simulink model "LQR_Active_suspension"  (R2024b)
settings: Solver=VariableStepAuto  StartTime=0.0  StopTime=10.0  RelTol=1e-3
values from neighbouring files (symbols this model uses):
  A = [ 0 1 0 -1 ... (first row only)    [param.m]
  a = 0.4    [param.m]
  B = [0  0 ... (first row only)    [param.m]
  C = [ 1 0 0 0 ... (first row only)    [param.m]
  D = [0 0 ... (first row only)    [param.m]
  F = 3    [param.m]
  K = lqr( A, B(:,2), Q, R )    [param.m]
libraries: eeGeneralControl x1
settings Model: Creator=rob  LastModifiedBy=rob

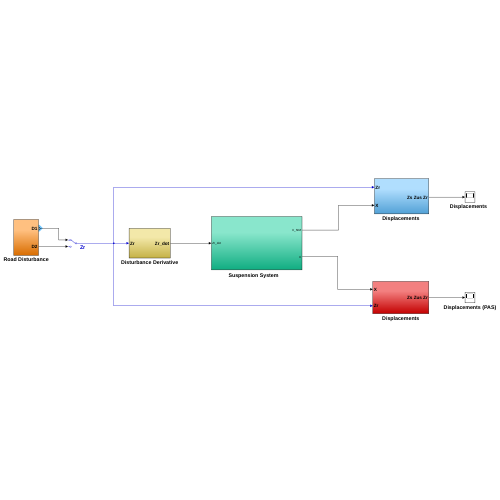
[thumbnail: Simulink's stored preview of the top-level diagram]
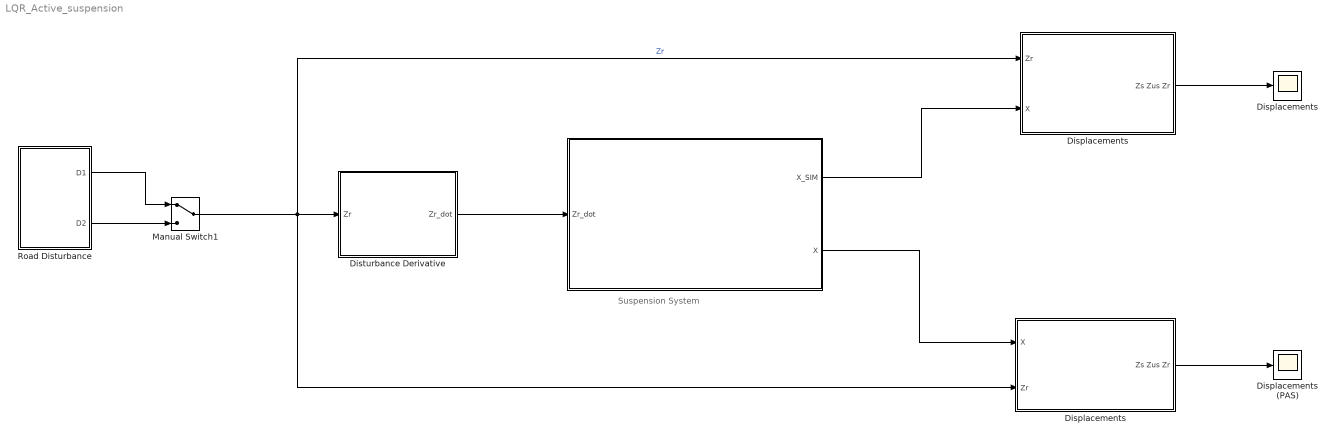
== system LQR_Active_suspension ==
  note: Suspension System
  " " : Subsystem
  Displacements : Subsystem
  "Displacements " : Subsystem
  "Displacements  " : Scope
  Displacements (PAS) : Scope
  Disturbance Derivative : Subsystem
  Manual Switch1 : ManualSwitch
  Road Disturbance : Subsystem
  wires:
  "Displacements "/1(Zs Zus Zr) -> "Displacements  "/1
  Road Disturbance/2(D2) -> Manual Switch1/2
  Road Disturbance/1(D1) -> Manual Switch1/1
  Manual Switch1/1 -> Disturbance Derivative/1(Zr), Displacements/2(Zr), "Displacements "/1(Zr)  "Zr"
  Displacements/1(Zs Zus Zr) -> Displacements (PAS)/1
  " "/2(X) -> Displacements/1(X)
  " "/1(X_SIM) -> "Displacements "/2(X)
  Disturbance Derivative/1(Zr_dot) -> " "/1(Zr_dot)

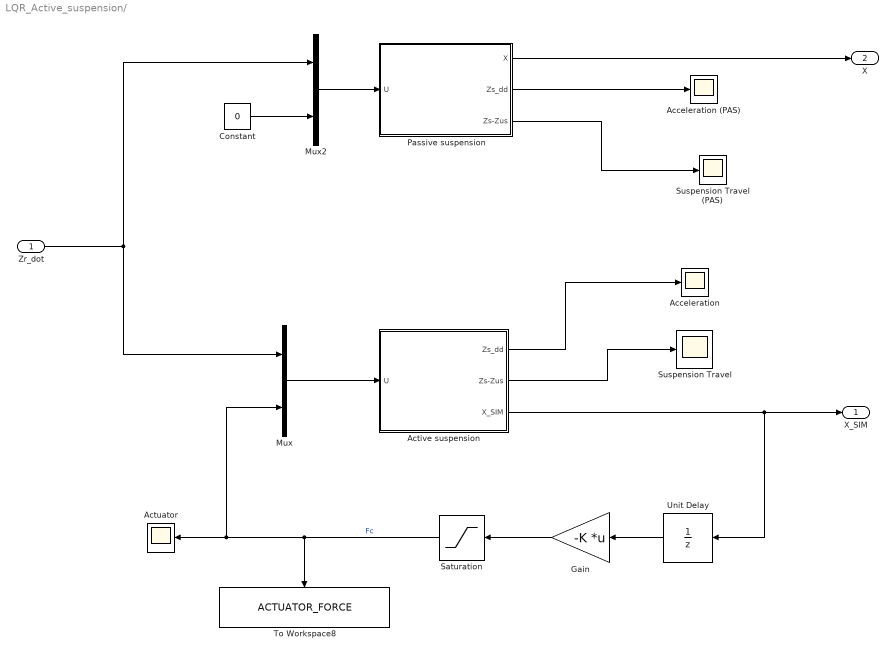
== system LQR_Active_suspension/  ==
  Zr_dot : Inport
  Acceleration : Scope
  Acceleration (PAS) : Scope
  Active suspension : Subsystem
  Actuator : Scope
  Constant : Constant  Value=0
  "Gain " : Gain  Gain=-K  Multiplication=Matrix(K*u)
  Mux : Mux  Inputs=2
  Mux2 : Mux  Inputs=2
  Passive suspension : Subsystem
  Saturation : Saturate  UpperLimit=45000  LowerLimit=-45000
  Suspension Travel : Scope
  Suspension Travel (PAS) : Scope
  To Workspace8 : ToWorkspace  VariableName=ACTUATOR_FORCE  SaveFormat=Timeseries  SampleTime=-1
  Unit Delay : UnitDelay  SampleTime=-1  HasFrameUpgradeWarning=on
  X_SIM : Outport
  X : Outport  Port=2
  wires:
  Active suspension/1(Zs_dd) -> Acceleration/1
  Mux/1 -> Active suspension/1(U)
  Zr_dot/1 -> Mux/1, Mux2/1
  Unit Delay/1 -> "Gain "/1
  Constant/1 -> Mux2/2
  Saturation/1 -> Mux/2, Actuator/1, To Workspace8/1  "Fc"
  "Gain "/1 -> Saturation/1
  Active suspension/3(X_SIM) -> X_SIM/1, Unit Delay/1
  Mux2/1 -> Passive suspension/1(U)
  Passive suspension/2(Zs_dd) -> Acceleration (PAS)/1
  Active suspension/2(Zs-Zus) -> Suspension Travel/1
  Passive suspension/3(Zs-Zus) -> Suspension Travel (PAS)/1
  Passive suspension/1(X) -> X/1

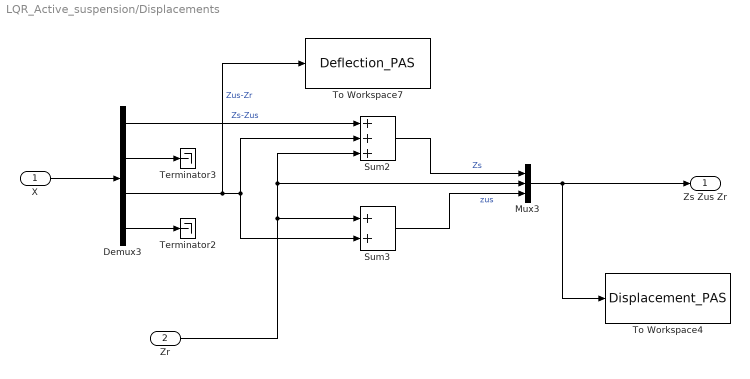
== system LQR_Active_suspension/Displacements ==
  X : Inport
  Zr : Inport  Port=2
  Demux3 : Demux
  Mux3 : Mux  Inputs=3
  Sum2 : Sum  Inputs=+++
  Sum3 : Sum
  Terminator2 : Terminator
  Terminator3 : Terminator
  To Workspace4 : ToWorkspace  VariableName=Displacement_PAS  SaveFormat=Timeseries  SampleTime=-1
  To Workspace7 : ToWorkspace  VariableName=Deflection_PAS  SaveFormat=Timeseries  SampleTime=-1
  Zs Zus Zr : Outport
  wires:
  Demux3/2 -> Terminator3/1
  Demux3/4 -> Terminator2/1
  Demux3/1 -> Sum2/1  "Zs-Zus"
  Demux3/3 -> To Workspace7/1, Sum3/2, Sum2/2  "Zus-Zr"
  Sum2/1 -> Mux3/1  "Zs"
  Sum3/1 -> Mux3/3  "zus"
  Mux3/1 -> Zs Zus Zr/1, To Workspace4/1
  Zr/1 -> Sum3/1, Mux3/2, Sum2/3
  X/1 -> Demux3/1

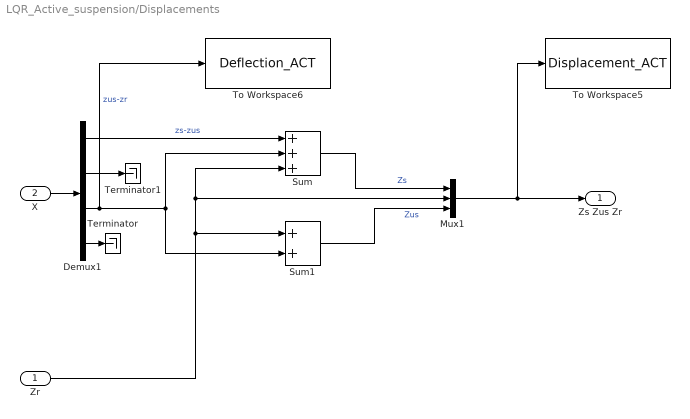
== system LQR_Active_suspension/Displacements  ==
  Zr : Inport
  X : Inport  Port=2
  Demux1 : Demux
  Mux1 : Mux  Inputs=3
  Sum : Sum  Inputs=+++
  Sum1 : Sum
  Terminator : Terminator
  Terminator1 : Terminator
  To Workspace5 : ToWorkspace  VariableName=Displacement_ACT  SaveFormat=Timeseries  SampleTime=-1
  To Workspace6 : ToWorkspace  VariableName=Deflection_ACT  SaveFormat=Timeseries  SampleTime=-1
  Zs Zus Zr : Outport
  wires:
  X/1 -> Demux1/1
  Demux1/2 -> Terminator1/1
  Demux1/4 -> Terminator/1
  Demux1/1 -> Sum/1  "zs-zus"
  Demux1/3 -> To Workspace6/1, Sum1/2, Sum/2  "zus-zr"
  Sum/1 -> Mux1/1  "Zs"
  Sum1/1 -> Mux1/3  "Zus"
  Mux1/1 -> Zs Zus Zr/1, To Workspace5/1
  Zr/1 -> Sum1/1, Mux1/2, Sum/3

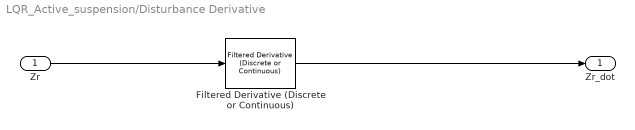
== system LQR_Active_suspension/Disturbance Derivative ==
  Zr : Inport
  Filtered Derivative (Discrete or Continuous) : eeGeneralControl/Filtered Derivative (Discrete or Continuous)  K=1  T=0.015  B=inf  A=-inf  minRatio=10  init_option=Inherited from block input  x0=0  Ts=-1
      settings: LibrarySourceBlock=|
      | ee_sl_lib/General Control/Filtered Derivative
      | (Discrete or Continuous)
  Zr_dot : Outport
  wires:
  Zr/1 -> Filtered Derivative (Discrete or Continuous)/1
  Filtered Derivative (Discrete or Continuous)/1 -> Zr_dot/1

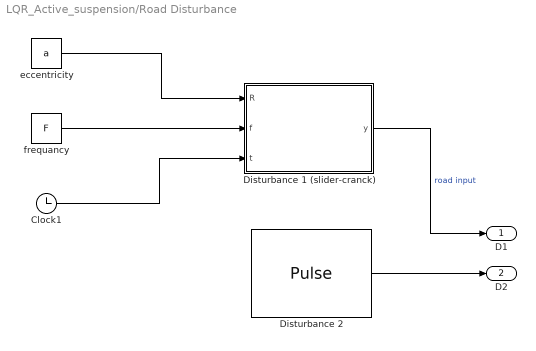
== system LQR_Active_suspension/Road Disturbance ==
  Clock1 : Clock
      settings: Decimation=Sim_Time
  Disturbance 1 (slider-cranck) : MATLAB Function  TreatAsAtomicUnit=on
  Disturbance 2 : DiscretePulseGenerator  PulseType=Time based  Amplitude=0.1  Period=6  PulseWidth=50  PhaseDelay=.1
  eccentricity : Constant  Value=a
  frequancy : Constant  Value=F
  D1 : Outport
  D2 : Outport  Port=2
  wires:
  Disturbance 2/1 -> D2/1
  eccentricity/1 -> Disturbance 1 (slider-cranck)/1(R)
  frequancy/1 -> Disturbance 1 (slider-cranck)/2(f)
  Clock1/1 -> Disturbance 1 (slider-cranck)/3(t)
  Disturbance 1 (slider-cranck)/1(y) -> D1/1  "road input"

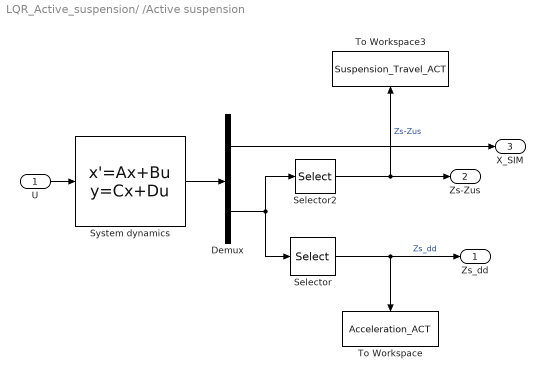
== system LQR_Active_suspension/ /Active suspension ==
  U : Inport
  Demux : Demux  Outputs=[4 2]
  Selector : Selector  InputPortWidth=2  IndexOptions=Index vector (dialog)  Indices=[2]  OutputSizes=1
  Selector2 : Selector  InputPortWidth=2  IndexOptions=Index vector (dialog)  Indices=[1]  OutputSizes=1
  System dynamics : StateSpace  A=A  B=B  C=cat(1,eye(4), C)  D=D  InitialCondition=0
  To Workspace : ToWorkspace  VariableName=Acceleration_ACT  SaveFormat=Timeseries  SampleTime=-1
  To Workspace3 : ToWorkspace  VariableName=Suspension_Travel_ACT  SaveFormat=Timeseries  SampleTime=-1
  Zs_dd : Outport
  Zs-Zus : Outport  Port=2
  X_SIM : Outport  Port=3
  wires:
  Demux/1 -> X_SIM/1
  System dynamics/1 -> Demux/1
  Demux/2 -> Selector2/1, Selector/1
  Selector/1 -> Zs_dd/1, To Workspace/1  "Zs_dd"
  Selector2/1 -> Zs-Zus/1, To Workspace3/1  "Zs-Zus"
  U/1 -> System dynamics/1

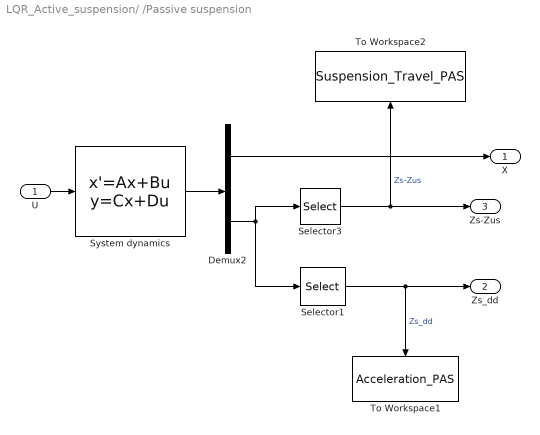
== system LQR_Active_suspension/ /Passive suspension ==
  U : Inport
  Demux2 : Demux  Outputs=[4 2]
  Selector1 : Selector  InputPortWidth=2  IndexOptions=Index vector (dialog)  Indices=[2]  OutputSizes=1
  Selector3 : Selector  InputPortWidth=2  IndexOptions=Index vector (dialog)  Indices=[1]  OutputSizes=1
  System dynamics : StateSpace  A=A  B=B  C=cat(1,eye(4), C)  D=D  InitialCondition=0
  To Workspace1 : ToWorkspace  VariableName=Acceleration_PAS  SaveFormat=Timeseries  SampleTime=-1
  To Workspace2 : ToWorkspace  VariableName=Suspension_Travel_PAS  SaveFormat=Timeseries  SampleTime=-1
  X : Outport
  Zs_dd : Outport  Port=2
  Zs-Zus : Outport  Port=3
  wires:
  System dynamics/1 -> Demux2/1
  Selector1/1 -> Zs_dd/1, To Workspace1/1  "Zs_dd"
  Demux2/2 -> Selector3/1, Selector1/1
  Selector3/1 -> Zs-Zus/1, To Workspace2/1  "Zs-Zus"
  U/1 -> System dynamics/1
  Demux2/1 -> X/1

== matlab function LQR_Active_suspension/Road Disturbance/Disturbance 1 (slider-cranck) ==
  data: y output; R input; f input; t input
function y = fcn(R,f,t)
% R eccentricity
% f frequancy 
% t time
omega = 2 * pi*f;
L=0.43; %length of connecting road
n=L/R;
theta = (omega * t*180)/pi;
x = R* ((1-cosd(theta+90)) + (n-sqrt(n^2 - sind(theta+90).^2)))-R*((1-cosd(90)) + (n-sqrt(n^2 - sind(90).^2)));y = x;
